simulink model "Assignment_2"  (R2020b)
settings: Solver=VariableStepAuto  StartTime=0.0  StopTime=100.0  RelTol=1e-3
values from neighbouring files (symbols this model uses):
  b = 270    [Values.m]
  K1 = 5800    [Values.m]
  K2 = 155000    [Values.m]
  M1 = 495    [Values.m]
  M2 = 40    [Values.m]
settings Model: Creator=Shantam Garg  LastModifiedBy=Shantam Garg

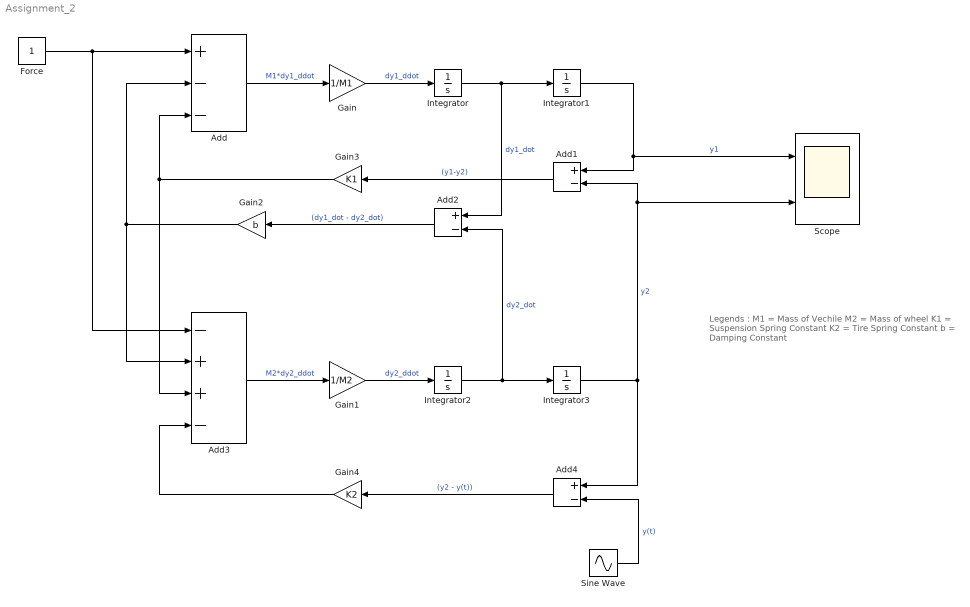
== system Assignment_2 ==
  note: Legends :
      | M1 = Mass of Vechile
      | M2 = Mass of wheel
      | K1 = Suspension Spring Constant
      | K2 = Tire Spring Constant
      | b = Damping Constant
  Add : Sum  Inputs=+--
  Add1 : Sum  Inputs=+-
  Add2 : Sum  Inputs=+-
  Add3 : Sum  Inputs=-++-
  Add4 : Sum  Inputs=+-
  Force : Constant
  Gain : Gain  Gain=1/M1
  Gain1 : Gain  Gain=1/M2
  Gain2 : Gain  Gain=b
  Gain3 : Gain  Gain=K1
  Gain4 : Gain  Gain=K2
  Integrator{,1..3} (4 alike) : Integrator
  Scope : Scope  NumInputPorts=2
  Sine Wave : Sin  Amplitude=2  Frequency=10  SampleTime=0
  wires:
  Add/1 -> Gain/1  "M1*dy1_ddot"
  Gain/1 -> Integrator/1  "dy1_ddot"
  Integrator/1 -> Add2/1, Integrator1/1  "dy1_dot"
  Gain1/1 -> Integrator2/1  "dy2_ddot"
  Integrator2/1 -> Add2/2, Integrator3/1  "dy2_dot"
  Integrator3/1 -> Add1/2, Scope/2, Add4/1  "y2"
  Integrator1/1 -> Add1/1, Scope/1  "y1"
  Add2/1 -> Gain2/1  "(dy1_dot - dy2_dot)"
  Gain2/1 -> Add3/2, Add/2
  Add1/1 -> Gain3/1  "(y1-y2)"
  Gain3/1 -> Add3/3, Add/3
  Add3/1 -> Gain1/1  "M2*dy2_ddot"
  Gain4/1 -> Add3/4
  Force/1 -> Add3/1, Add/1
  Sine Wave/1 -> Add4/2  "y(t)"
  Add4/1 -> Gain4/1  "(y2 - y(t))"
